simulink model "tcsmdl"  (Simulink 5.0)
settings: Solver=ode45  StartTime=0  StopTime=15  FixedStep=TSTEP  RelTol=1e-3
PreLoadFcn:
  | cd programs\simulink_par
  | Run_ft_bike
  | cd ..\..
libraries: Solver_SF x1, simulink_extras x1
settings Model: LastModifiedBy=ywata  ExtModeTrigMode=oneshot  ExtModeArmWhenConnect=off  SaveTime=off  SaveOutput=off  LimitDataPoints=off  BooleanDataType=off  RTWOptions="-aEnforceIntegerDowncast=1 -aFoldNonRolledExpr=1 -aInlineInvariantSignals=1 -aInlineParameters=0 -aLocalBlockOutputs=1 -aRollThreshold=5 -aZeroInternalMemoryAtStartup=1 -aZeroExternalMemoryAtStartup=1 -aInitFltsAndDblsToZero=1 -aGenerateReport=0 -aGenCodeOnly=0 -aRTWVerbose=1 -aIncludeHyperlinkInReport=0 -aLaunchReport=0 -aForceParamTrailComments=0 -aGenerateComments=1 -aIgnoreCustomStorageClasses=1 -aIncHierarchyInIds=0 -aMaxRTWIdLen=31 -aShowEliminatedStatements=0 -aPrefixModelToSubsysFcnNames=1 -aIncDataTypeInIds=0 -aInsertBlockDesc=0 -aSimulinkBlockComments=1 -aInlinedPrmAccess=\"Literals\"  -aSuppressErrorStatus=0 -aModelReferenceCompliant=1 -aSupportNonInlinedSFcns=1 -aSupportContinuousTime=1 -aSupportComplex=1 -aSupportNonFinite=1 -aSupportAbsoluteTime=1 -aTargetFcnLib=\"ansi_tfl_tmw.mat\" -aMultiInstanceERTCode=0 -aLogVarNameModifier=\"rt_\" -aIsPILTarget=0 -aCombineOutputUpdateFcns=0 -aGenerateASAP2=0 -aGenerateSampleERTMain=0 -aGenerateFullHeader=1 -aUtilityFuncGeneration=\"Auto\" -aIncludeFileDelimiter=\"Auto\" -aIncludeMdlTerminateFcn=1 -aPurelyIntegerCode=0 -aERTCustomFileBanners=0 -aRTWCAPIStates=0 -aRTWCAPIParams=0 -aRTWCAPISignals=0 -aMatFileLogging=1 -aGenFloatMathFcnCalls=\"ANSI_C\" -aExtModeMexFile=\"ext_comm\" -aExtModeTransport=0 -aExtModeStaticAllocSize=1000000 -aExtModeTesting=0 -aExtModeStaticAlloc=0 -aExtMode=0"

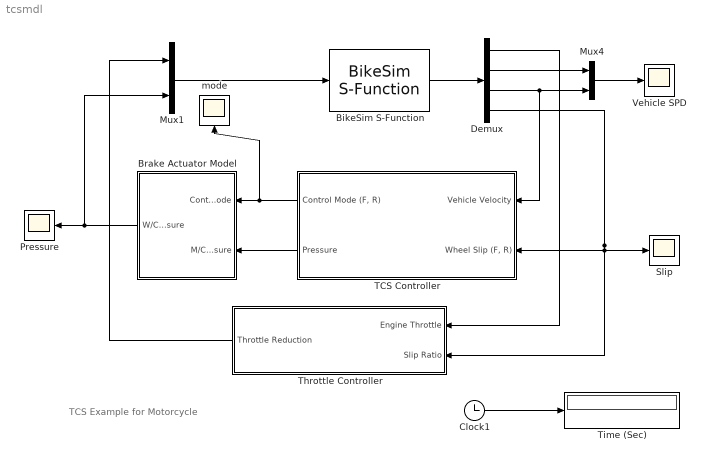
== system tcsmdl ==
  note: TCS Example for Motorcycle
  BikeSim S-Function : Solver_SF/BikeSim S-Function  Priority=1  AncestorBlock=Solver_SF/BikeSim S-Function  VehicleCode=i_i  SIMFILE=simfile
      settings: AttributesFormatString=Vehicle Code: %<VehicleCode>
  Brake Actuator Model : Subsystem  Orientation=left
  Clock1 : Clock
      settings: Decimation=10
  Demux : Demux  Outputs=[1 2 1 2 ]
  Mux1 : Mux  Inputs=2
  Mux4 : Mux  Inputs=2
  Pressure : Scope
      settings: TickLabels=on  TimeRange=15  YMin=-2  YMax=4  SaveName=ScopeData3  DataFormat=Array  SampleTime=100
  Slip : Scope
      settings: TickLabels=on  YMin=-1  YMax=2  SaveName=ScopeData4  DataFormat=Array  SampleTime=100
  TCS Controller : Subsystem  Orientation=left
  Throttle Controller : Subsystem  Orientation=left
  Time (Sec) : Display
  Vehicle SPD : Scope
      settings: YMin=-10  YMax=150
  mode : Scope
      settings: Orientation=up  TickLabels=on  YMin=-1  YMax=1  SaveName=ScopeData5  DataFormat=Array  SampleTime=100
  wires:
  BikeSim S-Function/1 -> Demux/1
  Mux1/1 -> BikeSim S-Function/1
  Demux/2 -> Mux4/1
  Demux/3 -> Mux4/2, TCS Controller/1(Vehicle Velocity)
  Mux4/1 -> Vehicle SPD/1
  Demux/4 -> TCS Controller/2("Wheel Slip (F, R)"), Slip/1, Throttle Controller/2(Slip Ratio)
  TCS Controller/1("Control Mode (F, R)") -> mode/1, Brake Actuator Model/1(Control Mode)
  TCS Controller/2(Pressure) -> Brake Actuator Model/2(M/C Pressure)
  Brake Actuator Model/1(W/C Pressure) -> Mux1/2, Pressure/1
  Demux/1 -> Throttle Controller/1(Engine Throttle)
  Throttle Controller/1(Throttle Reduction) -> Mux1/1
  Clock1/1 -> Time (Sec)/1

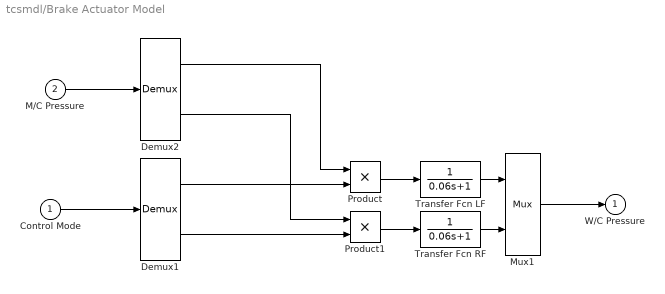
== system tcsmdl/Brake Actuator Model ==
  Control Mode : Inport
  M/C Pressure : Inport  Port=2
  Demux1 : Demux  Outputs=2
  Demux2 : Demux  Outputs=2
  Mux1 : Mux  Inputs=2
  Product : Product  SaturateOnIntegerOverflow=on  InputSameDT=on
  Product1 : Product  SaturateOnIntegerOverflow=on  InputSameDT=on
  Transfer Fcn LF : TransferFcn  Denominator=[0.06 1]
  Transfer Fcn RF : TransferFcn  Denominator=[0.06 1]
  W/C Pressure : Outport  InitialOutput=0
  wires:
  Mux1/1 -> W/C Pressure/1
  Control Mode/1 -> Demux1/1
  Product/1 -> Transfer Fcn LF/1
  Transfer Fcn LF/1 -> Mux1/1
  Product1/1 -> Transfer Fcn RF/1
  Transfer Fcn RF/1 -> Mux1/2
  Demux1/1 -> Product/2
  Demux1/2 -> Product1/2
  M/C Pressure/1 -> Demux2/1
  Demux2/1 -> Product/1
  Demux2/2 -> Product1/1

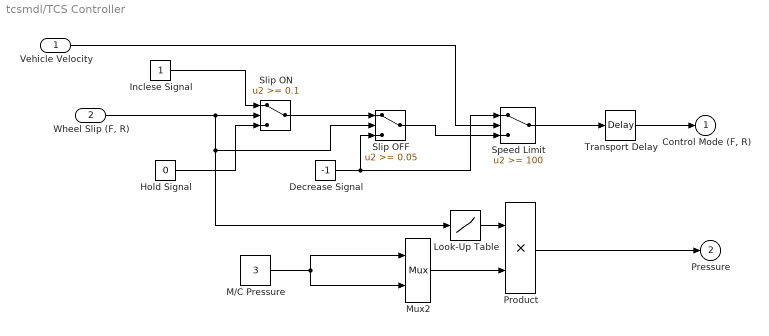
== system tcsmdl/TCS Controller ==
  Vehicle Velocity : Inport
  "Wheel Slip (F, R)" : Inport  Port=2
  Decrease Signal : Constant  Value=-1
  Hold Signal : Constant  Value=0
  Inclese Signal : Constant
  Look-Up Table : Lookup  InputValues=[-1,0,0.01,0.05,1,2]  OutputValues=[0,0,0.2,0.2,1.5,1.5]  SaturateOnIntegerOverflow=on
  M/C Pressure : Constant  Value=3
  Mux2 : Mux  Inputs=2
  Product : Product  SaturateOnIntegerOverflow=on  InputSameDT=on
  Slip OFF : Switch  Threshold=0.05  SaturateOnIntegerOverflow=on  InputSameDT=on
  Slip ON : Switch  Threshold=0.1  SaturateOnIntegerOverflow=on  InputSameDT=on
  Speed Limit : Switch  Threshold=100  SaturateOnIntegerOverflow=on  InputSameDT=on
  Transport Delay : TransportDelay  DelayTime=0.005
  "Control Mode (F, R)" : Outport  InitialOutput=0
  Pressure : Outport  Port=2  InitialOutput=0
  wires:
  Inclese Signal/1 -> Slip ON/1
  Slip ON/1 -> Slip OFF/1
  Hold Signal/1 -> Slip ON/3
  Speed Limit/1 -> Transport Delay/1
  Vehicle Velocity/1 -> Speed Limit/2
  "Wheel Slip (F, R)"/1 -> Slip ON/2, Slip OFF/2, Look-Up Table/1
  Slip OFF/1 -> Speed Limit/3
  Decrease Signal/1 -> Slip OFF/3, Speed Limit/1
  Transport Delay/1 -> "Control Mode (F, R)"/1
  Look-Up Table/1 -> Product/1
  Product/1 -> Pressure/1
  Mux2/1 -> Product/2
  M/C Pressure/1 -> Mux2/1, Mux2/2

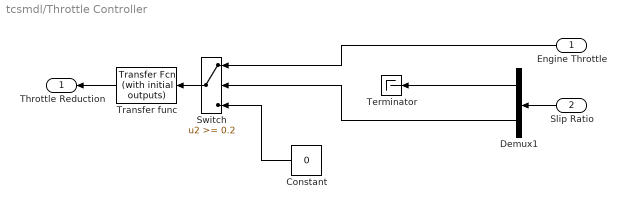
== system tcsmdl/Throttle Controller ==
  Engine Throttle : Inport  Orientation=left
  Slip Ratio : Inport  Orientation=left  Port=2
  Constant : Constant  Orientation=left  Value=0
  Demux1 : Demux  Orientation=left  Outputs=2
  Switch : Switch  Orientation=left  Threshold=0.2  SaturateOnIntegerOverflow=on  InputSameDT=on
  Terminator : Terminator
  Transfer func : simulink_extras/Additional Linear/Transfer Fcn (with initial outputs)  Orientation=left  N=[-10]  D="[1  1]"  Y0=0  U0=0
  Throttle Reduction : Outport  Orientation=left
  wires:
  Slip Ratio/1 -> Demux1/1
  Demux1/2 -> Switch/2
  Demux1/1 -> Terminator/1
  Constant/1 -> Switch/3
  Switch/1 -> Transfer func/1
  Engine Throttle/1 -> Switch/1
  Transfer func/1 -> Throttle Reduction/1
